simulink model "Det_sim"  (R2021a)
settings: Solver=VariableStepAuto  StartTime=0.0  StopTime=10.0  RelTol=1e-3
values from neighbouring files (symbols this model uses):
  F_input = reshape(F{1, 1}, [], 1)    [simulink_state_update_fn.m]
  g = 9.81    [ex02_dpa_Pendulum.m]    (also in simulink_state_update_fn.m; trace_state_update_fn.m; zCheck.m)
  L = 2    [ex02_dpa_Pendulum.m]    (also in simulink_state_update_fn.m; trace_state_update_fn.m; zCheck.m)
  m = (2689.8*L*pi*(D/2000)^2)    (= 0.844411972404)    [ex02_dpa_Pendulum.m]    (also in simulink_state_update_fn.m; trace_state_update_fn.m; zCheck.m)
  M = 1130.2    [ex02_dpa_Pendulum.m]    (also in simulink_state_update_fn.m; trace_state_update_fn.m; zCheck.m)
  nu = 6    [ex02_dpa_Pendulum.m]    (also in simulink_state_update_fn.m; trace_state_update_fn.m; zCheck.m)
  X1_0 = reshape(X{1, 1}, [], 1)    [simulink_state_update_fn.m]
  X2_0 = reshape(X{1, 2}, [], 1)    [simulink_state_update_fn.m]
settings Model: Creator=adekoyoa  LastModifiedBy=adekoyoa

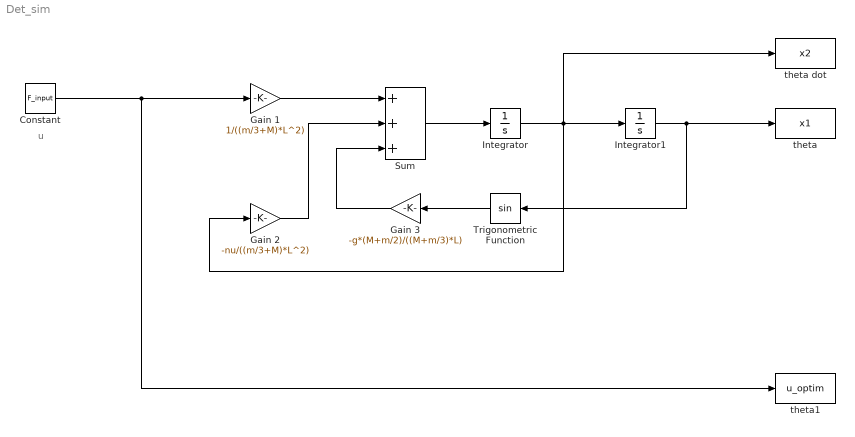
== system Det_sim ==
  note: u
  Constant : Constant  Value=F_input
  Gain 1 : Gain  Gain=1/((m/3+M)*L^2)
  Gain 2 : Gain  Gain=-nu/((m/3+M)*L^2)
  Gain 3 : Gain  Gain=-g*(M+m/2)/((M+m/3)*L)
  Integrator : Integrator  InitialCondition=X2_0
  Integrator1 : Integrator  InitialCondition=X1_0
  Sum : Sum  Inputs=+++
  Trigonometric Function : Trigonometry
  theta : ToWorkspace  VariableName=x1  SampleTime=-1
      settings: Save2DSignal=2-D array (concatenate along first dimension)
  theta dot : ToWorkspace  VariableName=x2  SampleTime=-1
      settings: Save2DSignal=2-D array (concatenate along first dimension)
  theta1 : ToWorkspace  VariableName=u_optim  SampleTime=-1
      settings: Save2DSignal=2-D array (concatenate along first dimension)
  wires:
  Integrator1/1 -> theta/1, Trigonometric Function/1
  Integrator/1 -> Gain 2/1, theta dot/1, Integrator1/1
  Trigonometric Function/1 -> Gain 3/1
  Sum/1 -> Integrator/1
  Gain 2/1 -> Sum/2
  Gain 3/1 -> Sum/3
  Gain 1/1 -> Sum/1
  Constant/1 -> theta1/1, Gain 1/1
